simulink model "Actuator_Model"  (R2025b)
settings: Solver=VariableStepAuto  StartTime=0.0  StopTime=10.0  RelTol=1e-3
undefined symbols (not defined in the file or in its folder): params
settings Model: Creator=samue  LastModifiedBy=samue

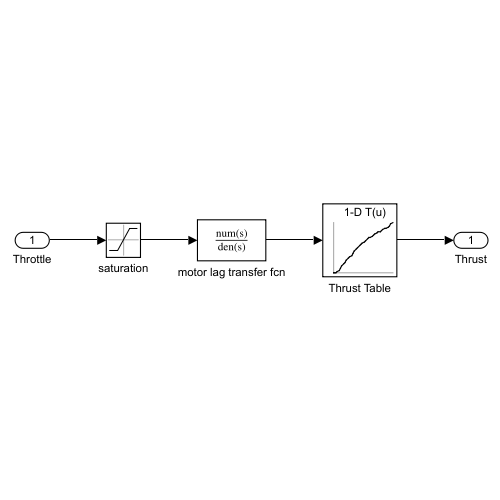
[thumbnail: Simulink's stored preview of the top-level diagram]
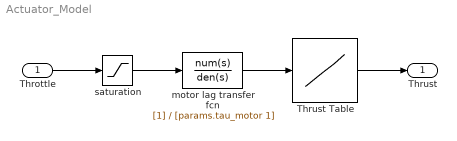
== system Actuator_Model ==
  Throttle : Inport
  Thrust Table : Lookup_n-D  NumberOfTableDimensions=1  BreakpointsForDimension1=params.throttle_array  Table=params.thrust_array  InternalRulePriority=Speed  RndMeth=Simplest
  motor lag transfer fcn : TransferFcn  Denominator=[params.tau_motor 1]
  saturation : Saturate  UpperLimit=100  LowerLimit=0
  Thrust : Outport
  wires:
  Throttle/1 -> saturation/1
  motor lag transfer fcn/1 -> Thrust Table/1
  Thrust Table/1 -> Thrust/1
  saturation/1 -> motor lag transfer fcn/1
